simulink model "Maso_priklad_04"  (R2022b)
settings: Solver=VariableStepAuto  StartTime=0.0  StopTime=3600.0  RelTol=1e-3
settings Model: Creator=honza  LastModifiedBy=honza

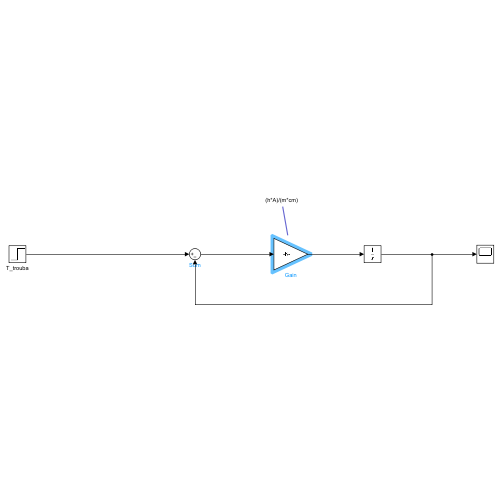
[thumbnail: Simulink's stored preview of the top-level diagram]
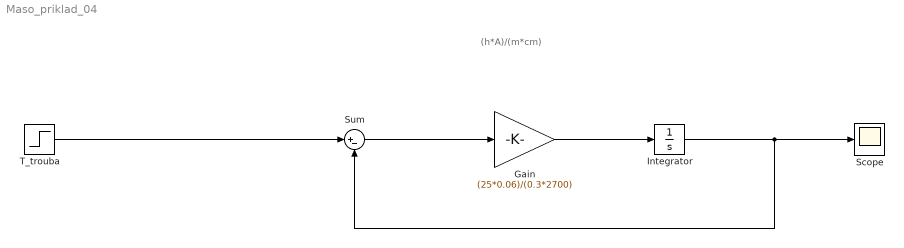
== system Maso_priklad_04 ==
  note: (h*A)/(m*cm)
  Gain : Gain  Gain=(25*0.06)/(0.3*2700)
  Integrator : Integrator  InitialCondition=5
  Scope : Scope
  Sum : Sum  Inputs=|+-
  T_trouba : Step  Time=0  After=200  SampleTime=0
  wires:
  Sum/1 -> Gain/1
  Integrator/1 -> Sum/2, Scope/1
  T_trouba/1 -> Sum/1
  Gain/1 -> Integrator/1
